simulink library "extended_kalman_filter_lib"  (R2016b)
settings: Solver=VariableStepAuto  StartTime=0.0  StopTime=10.0  RelTol=1e-3
undefined symbols (not defined in the file or in its folder): fsw_params
libraries: aerolibutil x1
settings Model: Creator=sexymathemagician  LastModifiedBy=Taylor

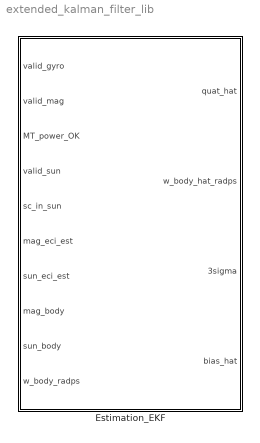
== system extended_kalman_filter_lib ==
  "Estimation_EKF " : Subsystem

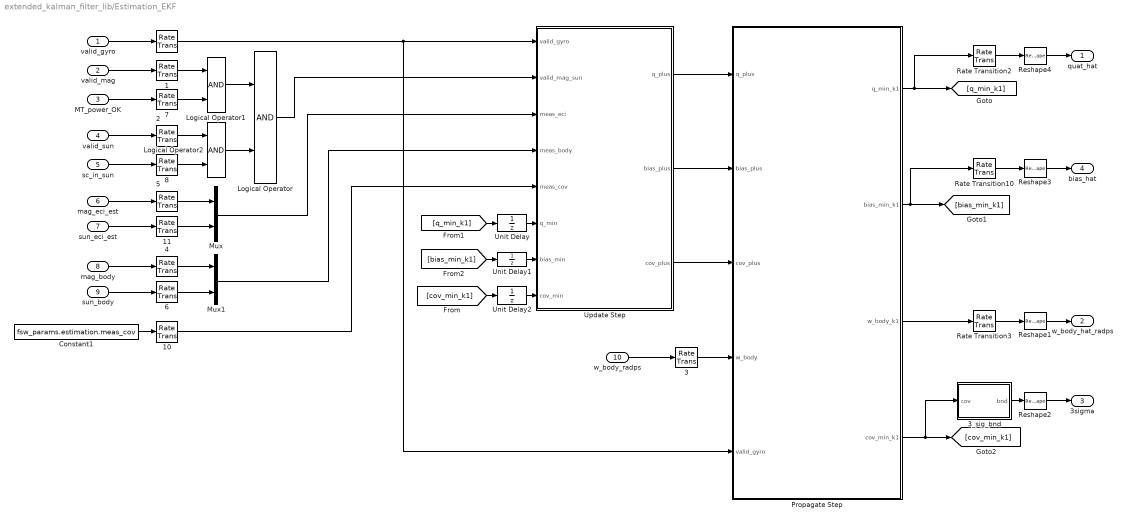
== system extended_kalman_filter_lib/Estimation_EKF  ==
  valid_gyro : Inport
  valid_mag : Inport  Port=2
  MT_power_OK : Inport  Port=3
  "valid_sun " : Inport  Port=4
  sc_in_sun : Inport  Port=5
  mag_eci_est : Inport  Port=6
  sun_eci_est : Inport  Port=7
  mag_body : Inport  Port=8
  sun_body : Inport  Port=9
  w_body_radps : Inport  Port=10
  " " : RateTransition  X0=fsw_params.estimation.ic.rt_valid_gyro  OutPortSampleTime=fsw_params.estimation.sample_time_s
  " 1" : RateTransition  X0=fsw_params.estimation.ic.rt_valid_mag  OutPortSampleTime=fsw_params.estimation.sample_time_s
  " 10" : RateTransition  X0=fsw_params.estimation.ic.rt_meas_cov  OutPortSampleTime=fsw_params.estimation.sample_time_s
  " 11" : RateTransition  X0=fsw_params.estimation.ic.rt_sun_eci_est  OutPortSampleTime=fsw_params.estimation.sample_time_s
  " 2" : RateTransition  X0=fsw_params.estimation.ic.rt_valid_sun  OutPortSampleTime=fsw_params.estimation.sample_time_s
  " 3" : RateTransition  X0=fsw_params.estimation.ic.rt_w_body_radps  OutPortSampleTime=fsw_params.estimation.sample_time_s
  " 4" : RateTransition  X0=fsw_params.estimation.ic.rt_mag_body  OutPortSampleTime=fsw_params.estimation.sample_time_s
  " 5" : RateTransition  X0=fsw_params.estimation.ic.rt_mag_eci_est  OutPortSampleTime=fsw_params.estimation.sample_time_s
  " 6" : RateTransition  X0=fsw_params.estimation.ic.rt_sun_body  OutPortSampleTime=fsw_params.estimation.sample_time_s
  " 7" : RateTransition  X0=fsw_params.estimation.ic.rt_mt_power_ok  OutPortSampleTime=fsw_params.estimation.sample_time_s
  " 8" : RateTransition  X0=fsw_params.estimation.ic.rt_sc_in_sun  OutPortSampleTime=fsw_params.estimation.sample_time_s
  "3_sig_bnd " : MATLAB Function  TreatAsAtomicUnit=on
  Constant1 : Constant  Value=fsw_params.estimation.meas_cov
  Logical Operator : Logic  AllPortsSameDT=off  OutDataTypeStr=boolean
  Logical Operator1 : Logic  AllPortsSameDT=off  OutDataTypeStr=boolean
  Logical Operator2 : Logic  AllPortsSameDT=off  OutDataTypeStr=boolean
  Mux : Mux  Inputs=2
  Mux1 : Mux  Inputs=2
  "Propagate Step " : Subsystem
  Rate Transition10 : RateTransition  X0=fsw_params.estimation.ic.bias_est_init
  Rate Transition2 : RateTransition  X0=fsw_params.estimation.ic.quat_est_init
  Rate Transition3 : RateTransition  X0=fsw_params.estimation.ic.rate_est_init
  Reshape{1..4} (4 alike) : Reshape  OutputDimensions=[3,1]
  Unit Delay : UnitDelay  InitialCondition=fsw_params.estimation.ic.quat_est_init  SampleTime=fsw_params.estimation.sample_time_s
  Unit Delay1 : UnitDelay  InitialCondition=fsw_params.estimation.ic.bias_est_init  SampleTime=fsw_params.estimation.sample_time_s
  Unit Delay2 : UnitDelay  InitialCondition=fsw_params.estimation.ic.error_cov  SampleTime=fsw_params.estimation.sample_time_s
  "Update Step " : Subsystem
  quat_hat : Outport
  w_body_hat_radps : Outport  Port=2
  3sigma : Outport  Port=3
  bias_hat : Outport  Port=4
  wires:
  "Update Step "/1(q_plus) -> "Propagate Step "/1(q_plus)
  "Update Step "/2(bias_plus) -> "Propagate Step "/2(bias_plus)
  "Update Step "/3(cov_plus) -> "Propagate Step "/3(cov_plus)
  valid_gyro/1 -> " "/1
  valid_mag/1 -> " 1"/1
  "valid_sun "/1 -> " 2"/1
  w_body_radps/1 -> " 3"/1
  mag_body/1 -> " 4"/1
  mag_eci_est/1 -> " 5"/1
  sun_body/1 -> " 6"/1
  sun_eci_est/1 -> " 11"/1
  Logical Operator/1 -> "Update Step "/2(valid_mag_sun)
  " 3"/1 -> "Propagate Step "/4(w_body)
  " 5"/1 -> Mux/1
  " 11"/1 -> Mux/2
  Mux/1 -> "Update Step "/3(meas_eci)
  " 4"/1 -> Mux1/1
  " 6"/1 -> Mux1/2
  Mux1/1 -> "Update Step "/4(meas_body)
  " 10"/1 -> "Update Step "/5(meas_cov)
  "Propagate Step "/1(q_min_k1) -> [q_min_k1], Rate Transition2/1
  "Propagate Step "/2(bias_min_k1) -> [bias_min_k1], Rate Transition10/1
  "Propagate Step "/3(w_body_k1) -> Rate Transition3/1
  " "/1 -> "Propagate Step "/5(valid_gyro), "Update Step "/1(valid_gyro)
  Reshape3/1 -> bias_hat/1
  Reshape2/1 -> 3sigma/1
  Reshape1/1 -> w_body_hat_radps/1
  Reshape4/1 -> quat_hat/1
  Rate Transition2/1 -> Reshape4/1
  Rate Transition3/1 -> Reshape1/1
  Rate Transition10/1 -> Reshape3/1
  "Propagate Step "/4(cov_min_k1) -> [cov_min_k1], "3_sig_bnd "/1(cov)
  "3_sig_bnd "/1(bnd) -> Reshape2/1
  [cov_min_k1] -> Unit Delay2/1
  Unit Delay2/1 -> "Update Step "/8(cov_min)
  [bias_min_k1] -> Unit Delay1/1
  Unit Delay1/1 -> "Update Step "/7(bias_min)
  [q_min_k1] -> Unit Delay/1
  Unit Delay/1 -> "Update Step "/6(q_min)
  Constant1/1 -> " 10"/1
  MT_power_OK/1 -> " 7"/1
  " 7"/1 -> Logical Operator1/2
  " 1"/1 -> Logical Operator1/1
  sc_in_sun/1 -> " 8"/1
  " 8"/1 -> Logical Operator2/2
  " 2"/1 -> Logical Operator2/1
  Logical Operator1/1 -> Logical Operator/1
  Logical Operator2/1 -> Logical Operator/2

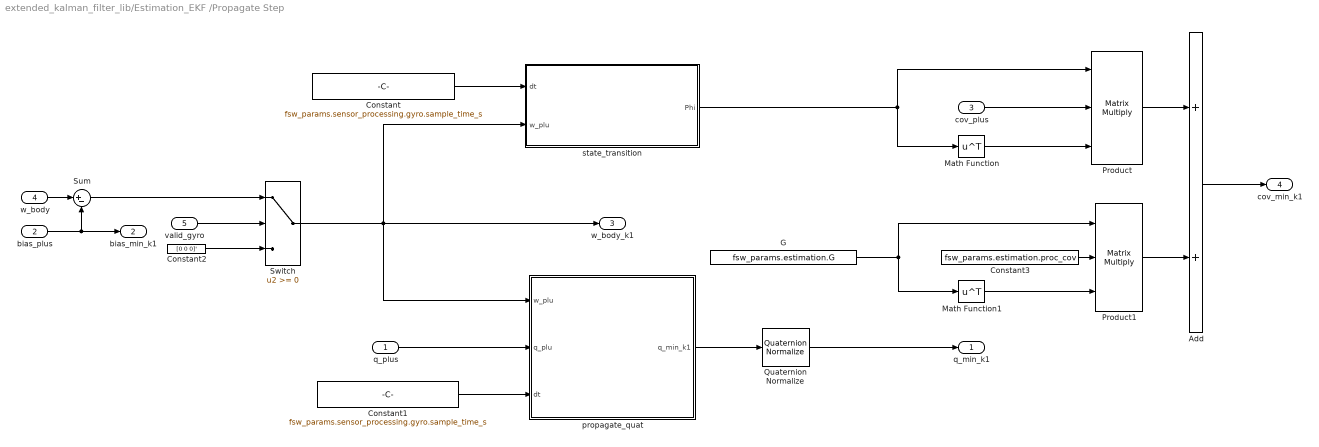
== system extended_kalman_filter_lib/Estimation_EKF /Propagate Step  ==
  q_plus : Inport
  bias_plus : Inport  Port=2
  cov_plus : Inport  Port=3
  w_body : Inport  Port=4
  valid_gyro : Inport  Port=5
  Add : Sum
  Constant : Constant  Value=fsw_params.sensor_processing.gyro.sample_time_s
  Constant1 : Constant  Value=fsw_params.sensor_processing.gyro.sample_time_s
  Constant2 : Constant  Value=[0 0 0]'
  Constant3 : Constant  Value=fsw_params.estimation.proc_cov
  G : Constant  Value=fsw_params.estimation.G
  Math Function : Math  Operator=transpose  SaturateOnIntegerOverflow=on
  Math Function1 : Math  Operator=transpose  SaturateOnIntegerOverflow=on
  Product : Product  Inputs=***  Multiplication=Matrix(*)  RndMeth=Zero
  Product1 : Product  Inputs=***  Multiplication=Matrix(*)  RndMeth=Zero
  Quaternion Normalize : aerolibutil/Quaternion Normalize
  Sum : Sum  Inputs=|+-
  Switch : Switch
  propagate_quat : MATLAB Function  TreatAsAtomicUnit=on
  state_transition : MATLAB Function  TreatAsAtomicUnit=on
  q_min_k1 : Outport
  bias_min_k1 : Outport  Port=2
  w_body_k1 : Outport  Port=3
  cov_min_k1 : Outport  Port=4
  wires:
  q_plus/1 -> propagate_quat/2(q_plu)
  Constant/1 -> state_transition/1(dt)
  Constant1/1 -> propagate_quat/3(dt)
  valid_gyro/1 -> Switch/2
  w_body/1 -> Sum/1
  bias_plus/1 -> bias_min_k1/1, Sum/2
  Switch/1 -> w_body_k1/1, propagate_quat/1(w_plu), state_transition/2(w_plu)
  propagate_quat/1(q_min_k1) -> Quaternion Normalize/1
  Quaternion Normalize/1 -> q_min_k1/1
  Product1/1 -> Add/2
  Product/1 -> Add/1
  Constant3/1 -> Product1/2
  Math Function1/1 -> Product1/3
  G/1 -> Product1/1, Math Function1/1
  cov_plus/1 -> Product/2
  Math Function/1 -> Product/3
  Add/1 -> cov_min_k1/1
  state_transition/1(Phi) -> Math Function/1, Product/1
  Constant2/1 -> Switch/3
  Sum/1 -> Switch/1

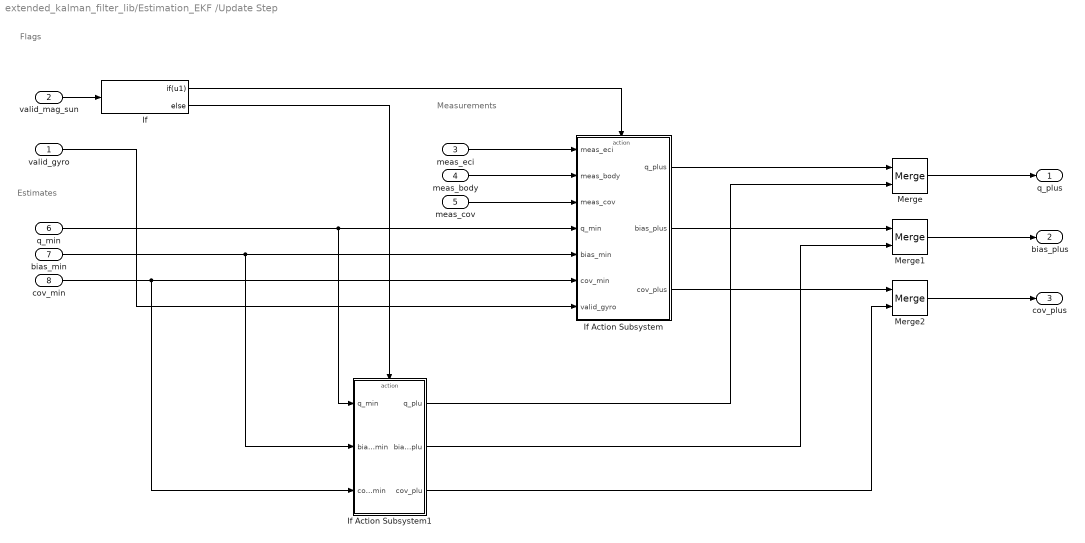
== system extended_kalman_filter_lib/Estimation_EKF /Update Step  ==
  note: Flags
  note: Estimates
  note: Measurements
  valid_gyro : Inport
  valid_mag_sun : Inport  Port=2
  meas_eci : Inport  Port=3
  meas_body : Inport  Port=4
  meas_cov : Inport  Port=5
  q_min : Inport  Port=6
  bias_min : Inport  Port=7
  cov_min : Inport  Port=8
  If : If  IfExpression=u1
  If Action Subsystem : Subsystem  TreatAsAtomicUnit=on
  If Action Subsystem1 : Subsystem  TreatAsAtomicUnit=on
  Merge : Merge
  Merge1 : Merge
  Merge2 : Merge
  q_plus : Outport
  bias_plus : Outport  Port=2
  cov_plus : Outport  Port=3
  wires:
  valid_mag_sun/1 -> If/1
  q_min/1 -> If Action Subsystem1/1(q_min), If Action Subsystem/4("q_min ")
  bias_min/1 -> If Action Subsystem1/2(bias_min), If Action Subsystem/5(bias_min)
  cov_min/1 -> If Action Subsystem1/3(cov_min), If Action Subsystem/6(cov_min)
  Merge/1 -> q_plus/1
  Merge1/1 -> bias_plus/1
  Merge2/1 -> cov_plus/1
  If Action Subsystem1/1(q_plu) -> Merge/2
  If Action Subsystem1/2(bias_plu) -> Merge1/2
  If Action Subsystem1/3(cov_plu) -> Merge2/2
  meas_eci/1 -> If Action Subsystem/1(meas_eci)
  meas_body/1 -> If Action Subsystem/2("meas_body ")
  meas_cov/1 -> If Action Subsystem/3(meas_cov)
  valid_gyro/1 -> If Action Subsystem/7(valid_gyro)
  If Action Subsystem/1(q_plus) -> Merge/1
  If Action Subsystem/2(bias_plus) -> Merge1/1
  If Action Subsystem/3(cov_plus) -> Merge2/1
  If/1 -> If Action Subsystem/Action
  If/2 -> If Action Subsystem1/Action

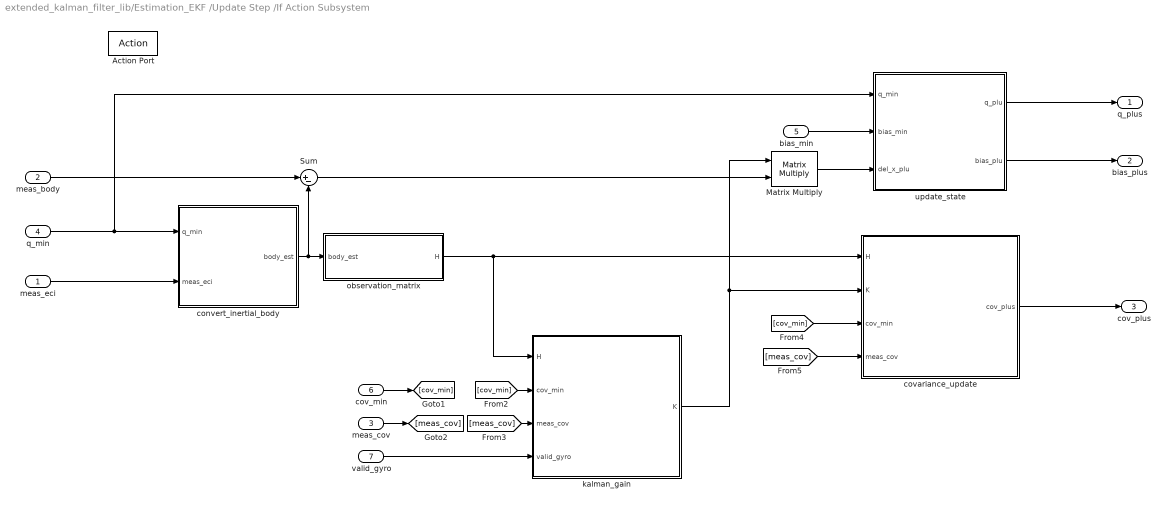
== system extended_kalman_filter_lib/Estimation_EKF /Update Step /If Action Subsystem ==
  meas_eci : Inport
  "meas_body " : Inport  Port=2
  meas_cov : Inport  Port=3
  "q_min " : Inport  Port=4
  bias_min : Inport  Port=5
  cov_min : Inport  Port=6
  valid_gyro : Inport  Port=7
  Action Port : ActionPort
  Matrix Multiply : Product  Multiplication=Matrix(*)
  Sum : Sum  Inputs=|+-
  convert_inertial_body : MATLAB Function  TreatAsAtomicUnit=on
  covariance_update : MATLAB Function  TreatAsAtomicUnit=on
  kalman_gain : MATLAB Function  TreatAsAtomicUnit=on
  observation_matrix : MATLAB Function  TreatAsAtomicUnit=on
  "update_state " : MATLAB Function  TreatAsAtomicUnit=on
  q_plus : Outport
  bias_plus : Outport  Port=2
  cov_plus : Outport  Port=3
  wires:
  convert_inertial_body/1(body_est) -> Sum/2, observation_matrix/1(body_est)
  meas_eci/1 -> convert_inertial_body/2(meas_eci)
  valid_gyro/1 -> kalman_gain/4(valid_gyro)
  observation_matrix/1(H) -> covariance_update/1(H), kalman_gain/1(H)
  "meas_body "/1 -> Sum/1
  kalman_gain/1(K) -> Matrix Multiply/1, covariance_update/2(K)
  covariance_update/1(cov_plus) -> cov_plus/1
  bias_min/1 -> "update_state "/2(bias_min)
  "update_state "/1(q_plu) -> q_plus/1
  "update_state "/2(bias_plu) -> bias_plus/1
  Sum/1 -> Matrix Multiply/2
  Matrix Multiply/1 -> "update_state "/3(del_x_plu)
  cov_min/1 -> [cov_min]
  [cov_min] -> kalman_gain/2(cov_min)
  meas_cov/1 -> [meas_cov]
  [meas_cov] -> kalman_gain/3(meas_cov)
  [cov_min] -> covariance_update/3(cov_min)
  [meas_cov] -> covariance_update/4(meas_cov)
  "q_min "/1 -> "update_state "/1(q_min), convert_inertial_body/1(q_min)

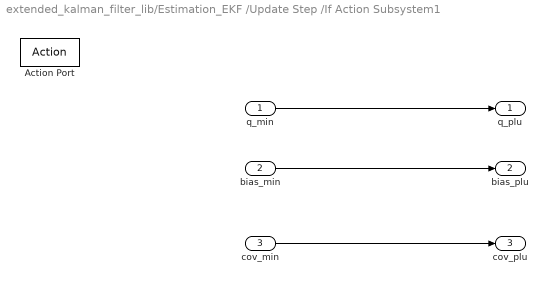
== system extended_kalman_filter_lib/Estimation_EKF /Update Step /If Action Subsystem1 ==
  q_min : Inport
  bias_min : Inport  Port=2
  cov_min : Inport  Port=3
  Action Port : ActionPort
  q_plu : Outport
  bias_plu : Outport  Port=2
  cov_plu : Outport  Port=3
  wires:
  q_min/1 -> q_plu/1
  bias_min/1 -> bias_plu/1
  cov_min/1 -> cov_plu/1

== matlab function extended_kalman_filter_lib/Estimation_EKF /Update Step /If Action Subsystem/convert_inertial_body ==
  data: q_min input; body_est output; meas_eci input
function body_est = convert_inertial_body(q_min,meas_eci)

rotation_matrix = att(q_min);
body_est = blkdiag(rotation_matrix,rotation_matrix)*meas_eci;

end

function dcm = att(q)
dcm = [q(1)^2 + q(2)^2 - q(3)^2 - q(4)^2,   2*(q(2)*q(3)+q(1)*q(4)),    2*(q(2)*q(4) - q(1)*q(3));
        2*(q(2)*q(3) - q(1)*q(4)),          q(1)^2-q(2)^2+q(3)^2-q(4)^2,    2*(q(3)*q(4) + q(1)*q(2));
        2*(q(2)*q(4)+q(1)*q(3)),            2*(q(3)*q(4)-q(1)*q(2)),        q(1)^2-q(2)^2-q(3)^2+q(4)^2];
end

== matlab function extended_kalman_filter_lib/Estimation_EKF /Update Step /If Action Subsystem/covariance_update ==
  data: H input; cov_plus output; K input; cov_min input; meas_cov input
function cov_plus = covariance_update(H,K,cov_min,meas_cov)


 KHI = (K*H - eye(6));
 cov_plus = KHI*cov_min*KHI' + K*meas_cov*K';


end

== matlab function extended_kalman_filter_lib/Estimation_EKF /Update Step /If Action Subsystem/kalman_gain ==
  data: H input; K output; cov_min input; meas_cov input; valid_gyro input
function K = kalman_gain(H,cov_min,meas_cov,valid_gyro)

K = cov_min*H'/(H*cov_min*H' + meas_cov);

% zero off part of gain if gyro reading is invalid

if valid_gyro == 0
    K(4:6,:) = zeros(3,6);
end


end

== matlab function extended_kalman_filter_lib/Estimation_EKF /Update Step /If Action Subsystem/observation_matrix ==
  data: body_est input; H output
function H = observation_matrix(body_est)

H = [  skew(body_est(1:3))     zeros(3);
       skew(body_est(4:6))     zeros(3)];

end

function S = skew(v)
S = [0  -v(3)   v(2);
    v(3)    0   -v(1);
    -v(2)   v(1)    0];
end

== matlab function extended_kalman_filter_lib/Estimation_EKF /Update Step /If Action Subsystem/update_state  ==
  data: q_min input size=4; q_plu output size=4; bias_min input size=3; del_x_plu input size=6; bias_plu output size=3
function [q_plu,bias_plu] = update_state(q_min,bias_min,del_x_plu)
%#codegen

% select out bias
bias_plu = bias_min + del_x_plu(4:6);

q_plu = quat_update(del_x_plu(1:3),q_min);
q_plu = q_plu/norm(q_plu);

end


function q_hat_pk = quat_update(del_apk, q_hat_mk)
%#codegen

% this has a sqrt error if del_apk is too large, i.e. small angle
% approximation doesn't hold
%q_hat_pk = quat_multiply([sqrt(1-norm(del_apk/2)); del_apk/2], q_hat_mk);

% the following two equations are equivalent; the first is probably a bit
% more computationally cheaper
q_hat_pk = quat_multiply([1; del_apk/2], q_hat_mk);
%q_hat_pk = q_hat_mk + 0.5*xi_matrix(q_hat_mk)*del_apk;
end

function xi = xi_matrix(q)
%#codegen

q1 = q(1);
v = q(2:4);

xi = zeros(4,3);
xi(1,:) = -[v(1) v(2) v(3)];
xi(2:4,:) = q1*eye(3) + skew(v);

end

function q2 = quat_multiply(dq,q1)
%#codegen

q2 = quatmultiply(q1',dq')';
end

function S = skew(v)
%#codegen
S = [0  -v(3)   v(2);
    v(3)    0   -v(1);
    -v(2)   v(1)    0];
end

== matlab function extended_kalman_filter_lib/Estimation_EKF /Propagate Step /state_transition ==
  data: dt input; w_plu input; Phi output
function Phi = state_transition(dt,w_plu)

Phi = state_transition_matrix(w_plu,dt);

end

function phi = state_transition_matrix(w, dt)
%#codegen

w_n = norm(w);
w_skew = skew(w);

if w_n < 1e-14
    phi = [ eye(3) -eye(3)*dt;
            zeros(3,3) eye(3)];
else
    Phi_11 = eye(3) - w_skew*sin(w_n*dt)/w_n + w_skew^2*(1 - cos(w_n*dt))/w_n^2;
    
    Phi_12 = w_skew*(1 - cos(w_n*dt))/w_n^2 - eye(3)*dt - w_skew^2*(w_n*dt - sin(w_n*dt))/w_n^3;
    
    Phi_21 = zeros(3,3);
    
    Phi_22 = eye(3);
    
    phi = [ Phi_11 Phi_12;
            Phi_21 Phi_22];
end
end

function S = skew(v)
S = [0  -v(3)   v(2);
    v(3)    0   -v(1);
    -v(2)   v(1)    0];
end

== matlab function extended_kalman_filter_lib/Estimation_EKF /Propagate Step /propagate_quat ==
  data: w_plu input; q_min_k1 output; q_plu input; dt input
function q_min_k1 = propagate_quat(w_plu,q_plu,dt)
%#codegen

q_min_k1 = omega_matrix(w_plu,dt)*q_plu;

end

function omega = omega_matrix(w, dt)
%#codegen
w_n = norm(w);

if w_n < 1e-14
    Psi = 0*w;
else
    Psi = sin(1/2*w_n*dt)/w_n*w;
end

Psi_skew = skew(Psi);

omega = [cos(1/2*w_n*dt)*eye(3) - Psi_skew      Psi;
        -Psi'                                   cos(1/2*w_n*dt)];

T = [zeros(3,1) eye(3);
    1       zeros(1,3)];

omega = T'*omega*T;
end

function S = skew(v)
%#codegen
S = [0  -v(3)   v(2);
    v(3)    0   -v(1);
    -v(2)   v(1)    0];
end

== matlab function extended_kalman_filter_lib/Estimation_EKF /3_sig_bnd  ==
  data: cov input; bnd output
function bnd =  three_sig_bnd(cov)

bnd = cov;
